simulink model "simuintro"  (R2021a)
settings: Solver=VariableStepAuto  StartTime=0.0  StopTime=10.0  RelTol=1e-3
settings Model: Creator=PRAVEEN MITTAL  LastModifiedBy=PRAVEEN MITTAL

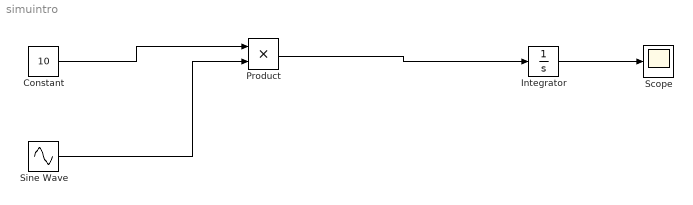
== system simuintro ==
  Constant : Constant  Value=10
  Integrator : Integrator
  Product : Product
  Scope : Scope
  Sine Wave : Sin  SampleTime=0
  wires:
  Integrator/1 -> Scope/1
  Constant/1 -> Product/1
  Product/1 -> Integrator/1
  Sine Wave/1 -> Product/2
